simulink model "prueba_de_fricciones"  (R2014a)
settings: Solver=ode23t  StartTime=0.0  StopTime=2  RelTol=1e-3
libraries: nesl_utility x12, fl_lib x6, Fricciones x3, simulink x1
settings Model: Creator=Sebastian  LastModifiedBy=Sebastian

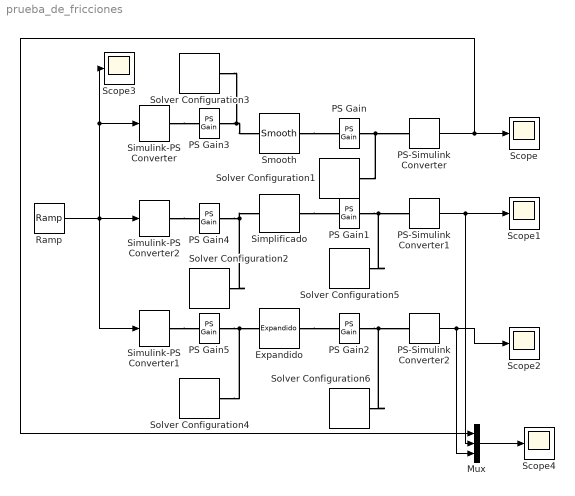
== system prueba_de_fricciones ==
  Expandido : Fricciones/Expandido  SystemSampleTime=-1
  Mux : Mux  Inputs=3
  PS Gain{,1..5} (6 alike) : fl_lib/Physical Signals/Functions/PS Gain  gain=1
  PS-Simulink Converter : nesl_utility/PS-Simulink Converter  PhysicalDomain=network_engine_domain  SubClassName=ps_output  LeftPortType=input  RightPortType=output  PseudoPeriodic=off  Frequencies=[]  Unit=1  AffineConversion=off
  PS-Simulink Converter1 : nesl_utility/PS-Simulink Converter  PhysicalDomain=network_engine_domain  SubClassName=ps_output  LeftPortType=input  RightPortType=output  PseudoPeriodic=off  Frequencies=[]  Unit=1  AffineConversion=off
  PS-Simulink Converter2 : nesl_utility/PS-Simulink Converter  PhysicalDomain=network_engine_domain  SubClassName=ps_output  LeftPortType=input  RightPortType=output  PseudoPeriodic=off  Frequencies=[]  Unit=1  AffineConversion=off
  Ramp : simulink/Sources/Ramp  slope=3  start=0  X0=-3
  Scope{,1..4} (5 alike) : Scope
      Scope settings: YMin=-0.11  YMax=0.005
      Scope1 settings: YMin=-0.11  YMax=0.005
      Scope2 settings: YMin=-0.11  YMax=0.005  SaveName=ScopeData2
      Scope3 settings: YMin=-0.11  YMax=0.005  SaveName=ScopeData3
      Scope4 settings: YMin=-0.11  YMax=0.005  SaveName=ScopeData4
  Simplificado : Fricciones/Simplificado
  Simulink-PS Converter : nesl_utility/Simulink-PS Converter  PhysicalDomain=network_engine_domain  SubClassName=ps_input  LeftPortType=input  RightPortType=output  PseudoPeriodic=off  Frequencies=[]  NoiseDistribution=none  NoiseParameters=[]  Unit=1  AffineConversion=off  InputFiltering=off  SimscapeFilterOrder=1  InputFilterTimeConstant=0.001  UdotUserProvided=1
  Simulink-PS Converter1 : nesl_utility/Simulink-PS Converter  PhysicalDomain=network_engine_domain  SubClassName=ps_input  LeftPortType=input  RightPortType=output  PseudoPeriodic=off  Frequencies=[]  NoiseDistribution=none  NoiseParameters=[]  Unit=1  AffineConversion=off  InputFiltering=off  SimscapeFilterOrder=1  InputFilterTimeConstant=0.001  UdotUserProvided=1
  Simulink-PS Converter2 : nesl_utility/Simulink-PS Converter  PhysicalDomain=network_engine_domain  SubClassName=ps_input  LeftPortType=input  RightPortType=output  PseudoPeriodic=off  Frequencies=[]  NoiseDistribution=none  NoiseParameters=[]  Unit=1  AffineConversion=off  InputFiltering=off  SimscapeFilterOrder=1  InputFilterTimeConstant=0.001  UdotUserProvided=1
  Smooth : Fricciones/Smooth  SystemSampleTime=-1
  Solver Configuration{1..6} (6 alike) : nesl_utility/Solver Configuration  PhysicalDomain=network_engine_domain  SubClassName=solver  LeftPortType=input  RightPortType=generic  Accelerate=off  Tones=[]  Harmonics=[]  SimulateNoise=off  Profile=off  UseLocalSampling=off  EnableSwitchedLinearOptims=on  FrequencyDomain=off  UseCCode=off  RelTol=0.001  AbsTol=1e-06  MinStep=1e-09  ToWorkspace=off  DoDC=on  ResidualTolerance=1e-09  UseLocalSolver=off  LocalSolverChoice=NE_BACKWARD_EULER_ADVANCER  LocalSolverSampleTime=0.0005  DoFixedCost=off  MaxNonlinIter=30  MaxModeIter=2  LinearAlgebra=Full  DelaysMemoryBudget=2048  AutomaticFiltering=on  FilteringTimeConstant=0.001
  wires:
  PS-Simulink Converter/1 -> Mux/1, Scope/1
  PS-Simulink Converter1/1 -> Mux/2, Scope1/1
  PS-Simulink Converter2/1 -> Mux/3, Scope2/1
  Ramp/1 -> Simulink-PS Converter1/1, Scope3/1, Simulink-PS Converter/1, Simulink-PS Converter2/1
  Mux/1 -> Scope4/1
  connections:
  Solver Configuration1/RConn1 -- PS-Simulink Converter/LConn1 -- PS Gain/RConn1
  Smooth/LConn1 -- PS Gain/LConn1
  Simplificado/LConn1 -- PS Gain1/LConn1
  PS Gain1/RConn1 -- Solver Configuration5/RConn1 -- PS-Simulink Converter1/LConn1
  Expandido/LConn1 -- PS Gain2/LConn1
  PS Gain2/RConn1 -- Solver Configuration6/RConn1 -- PS-Simulink Converter2/LConn1
  Simulink-PS Converter/RConn1 -- PS Gain3/LConn1
  PS Gain3/RConn1 -- Solver Configuration3/RConn1 -- Smooth/RConn1
  Simulink-PS Converter2/RConn1 -- PS Gain4/LConn1
  PS Gain4/RConn1 -- Simplificado/RConn1 -- Solver Configuration2/RConn1
  Simulink-PS Converter1/RConn1 -- PS Gain5/LConn1
  PS Gain5/RConn1 -- Solver Configuration4/RConn1 -- Expandido/RConn1
